simulink model "OSCILOS_Sim_lin"  (R2015a)
settings: Solver=ode3  StartTime=0.0  StopTime=0.5  FixedStep=dt  RelTol=1e-3
model workspace: external: MATLAB File /Users/amorgans/Documents/amorgans/OSCILOS/OSCILOS_SIM/parameters.m (data not in the file)
values from neighbouring files (symbols this model uses):
  dt = 10^-5    (= 1e-05)    [parameters.m]
libraries: OSCILOS_SIM x3
settings Model: CovSFcnEnable=off  Creator=Maxi  LastModifiedBy=amorgans
settings DebuggingCC: SolverPrmCheckMsg=warning

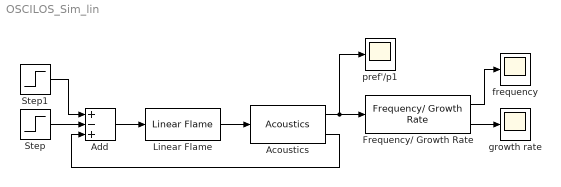
== system OSCILOS_Sim_lin ==
  Acoustics : OSCILOS_SIM/Acoustics  SystemSampleTime=-1
  Add : Sum  Inputs=+-+
  Frequency/ Growth Rate : OSCILOS_SIM/Frequency// Growth Rate  SystemSampleTime=-1
  Linear Flame : OSCILOS_SIM/Linear Flame  SystemSampleTime=-1
  Step : Step  Time=dt  SampleTime=0
  Step1 : Step  Time=0  SampleTime=0
  frequency : Scope
      settings: SaveName=ScopeData2
  growth rate : Scope
  pref'/p1 : Scope
  wires:
  Linear Flame/1 -> Acoustics/1
  Add/1 -> Linear Flame/1
  Acoustics/2 -> Add/3
  Step/1 -> Add/2
  Step1/1 -> Add/1
  Acoustics/1 -> pref'/p1/1, Frequency/ Growth Rate/1
  Frequency/ Growth Rate/2 -> growth rate/1
  Frequency/ Growth Rate/1 -> frequency/1
